simulink model "three_phase_topology"  (Simulink 8.5)
settings: Solver=ode45  StartTime=0.0  StopTime=10.0  MaxStep=0.0001  MinStep=0.00001  RelTol=1e-3
libraries: powerlib x37
settings Model: Creator=SELVA  LastModifiedBy=SELVA SAM  CovSFcnEnable=off
settings DataIOCC: SignalLoggingSaveFormat=Dataset
settings OptimizationCC: ExpressionDepthLimit=128
settings DebuggingCC: UnderspecifiedInitializationDetection=Simplified  MergeDetectMultiDrivingBlocksExec=error  SolverPrmCheckMsg=warning  FcnCallInpInsideContextMsg=EnableAllAsError  StateNameClashWarn=none
settings GRTTargetCC: CombineOutputUpdateFcns=on  GRTInterface=off
settings ConfigurationSet: Description=SimMechanics 2G

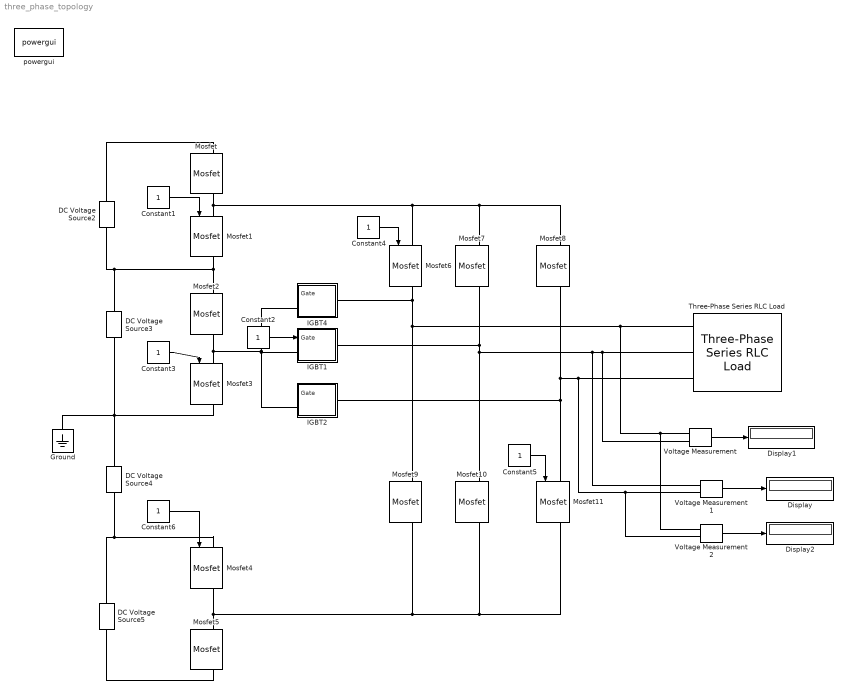
== system three_phase_topology ==
  Constant{1..6} (6 alike) : Constant
  DC Voltage Source{2..5} (4 alike) : powerlib/Electrical Sources/DC Voltage Source  Amplitude=600  Measurements=None
  Display : Display
  Display1 : Display
  Display2 : Display
  Ground : powerlib/Elements/Ground  LConnTagsString=a
  IGBT1 : Subsystem
  IGBT2 : Subsystem
  IGBT4 : Subsystem
  Mosfet{,1..11} (12 alike) : powerlib/Power Electronics/Mosfet  Ron=0.1  Lon=0  Rd=0.01  Vfd=0  IC=0  Rs=1e5  Cs=inf  Measurements=on
  Three-Phase Series RLC Load : powerlib/Elements/Three-Phase Series RLC Load  LConnTagsString=A|B|C  Configuration=Y (grounded)  NominalVoltage=400  NominalFrequency=50  ActivePower=1000  InductivePower=0  CapacitivePower=0  Measurements=None  LoadType=constant Z
  Voltage Measurement : powerlib/Measurements/Voltage Measurement  PhasorSimulation=off  OutputType=Complex  PSBequivalent=0
  Voltage Measurement1 : powerlib/Measurements/Voltage Measurement  PhasorSimulation=off  OutputType=Complex  PSBequivalent=0
  Voltage Measurement2 : powerlib/Measurements/Voltage Measurement  PhasorSimulation=off  OutputType=Complex  PSBequivalent=0
  powergui : powerlib/powergui  Priority=1  SimulationMode=Discrete  SolverType=Tustin/Backward Euler (TBE)  SampleTime=50e-6  frequency=60  SPID=off  DisableSnubberDevices=off  DisableRonSwitches=off  DisableVfSwitches=off  SwTol=0  DisplayEquations=off  Interpol=off  methode=off  Ts=100  frequencyindice=0  Pbase=100e6  ErrMax=1e-4  Iterations=50  UnitsV=kV  UnitsW=MW  FunctionMessages=off  echomessages=off  HookPort=off  EnableUseOfTLC=off  x0status=blocks  RestoreLinks=warning  ResistiveCurrentMeasurement=off  Frange=[0:2:500]  Ylog=off  Xlog=on  ShowGrid=off  save=off  variable=ZData  structure=0  ZoomFFT=off  StartTime=0.0  cycles=1  DisplayStyle=1  fundamental=60  FreqAxis=off  MaxFrequency=1000  frequencyindicesteady=1  RmsSteady=1  display=off
  wires:
  ? -> IGBT4/1(Gate)
  Constant2/1 -> IGBT1/1(Gate)
  ? -> IGBT2/1(Gate)
  Constant3/1 -> Mosfet3/1
  Constant4/1 -> Mosfet6/1
  Constant5/1 -> Mosfet11/1
  Constant1/1 -> Mosfet1/1
  Constant6/1 -> Mosfet4/1
  Voltage Measurement/1 -> Display1/1
  Voltage Measurement1/1 -> Display/1
  Voltage Measurement2/1 -> Display2/1
  connections:
  Mosfet3/LConn1 -- IGBT4/LConn1 -- IGBT2/LConn1 -- IGBT1/LConn1 -- Mosfet2/RConn1
  Mosfet2/LConn1 -- DC Voltage Source2/LConn1 -- DC Voltage Source3/RConn1 -- Mosfet1/RConn1
  DC Voltage Source2/RConn1 -- Mosfet/LConn1
  Ground/LConn1 -- DC Voltage Source4/RConn1 -- DC Voltage Source3/LConn1 -- Mosfet3/RConn1
  Mosfet4/LConn1 -- DC Voltage Source5/RConn1 -- DC Voltage Source4/LConn1
  Mosfet11/RConn1 -- Mosfet4/RConn1 -- Mosfet5/LConn1 -- Mosfet9/RConn1 -- Mosfet10/RConn1
  DC Voltage Source5/LConn1 -- Mosfet5/RConn1
  Mosfet11/LConn1 -- Voltage Measurement2/LConn2 -- Voltage Measurement1/LConn2 -- Three-Phase Series RLC Load/LConn3 -- Mosfet8/RConn1 -- IGBT2/RConn1
  Mosfet10/LConn1 -- Voltage Measurement1/LConn1 -- Voltage Measurement/LConn2 -- Three-Phase Series RLC Load/LConn2 -- Mosfet7/RConn1 -- IGBT1/RConn1
  Mosfet6/RConn1 -- Voltage Measurement2/LConn1 -- Voltage Measurement/LConn1 -- Three-Phase Series RLC Load/LConn1 -- Mosfet9/LConn1 -- IGBT4/RConn1
  Mosfet1/LConn1 -- Mosfet7/LConn1 -- Mosfet8/LConn1 -- Mosfet6/LConn1 -- Mosfet/RConn1

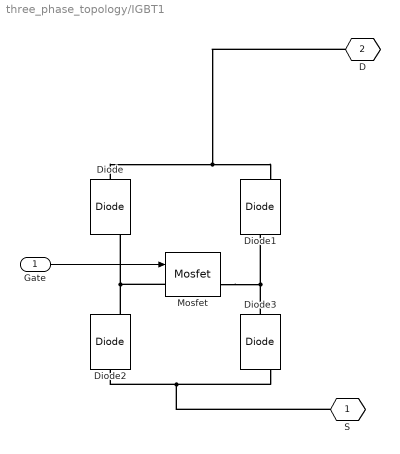
== system three_phase_topology/IGBT1 ==
  Gate : Inport
  Diode{,1..3} (4 alike) : powerlib/Power Electronics/Diode  Ron=0.001  Lon=0  Vf=0.8  IC=0  UseSnubber=off  Rs=500  Cs=250e-9  Measurements=on
  Mosfet : powerlib/Power Electronics/Mosfet  Ron=0.1  Lon=0  Rd=0.01  Vfd=0  IC=0  Rs=1e5  Cs=inf  Measurements=on
  S : PMIOPort  Port=1  Side=Left
  D : PMIOPort  Port=2  Side=Right
  wires:
  Gate/1 -> Mosfet/1
  connections:
  D/RConn1 -- Diode/LConn1 -- Diode1/RConn1
  S/RConn1 -- Diode3/RConn1 -- Diode2/LConn1
  Mosfet/RConn1 -- Diode3/LConn1 -- Diode1/LConn1
  Mosfet/LConn1 -- Diode2/RConn1 -- Diode/RConn1

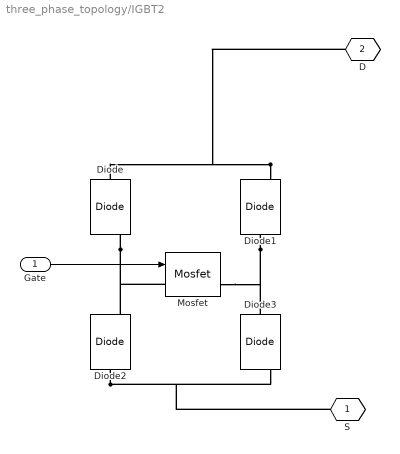
== system three_phase_topology/IGBT2 ==
  Gate : Inport
  Diode{,1..3} (4 alike) : powerlib/Power Electronics/Diode  Ron=0.001  Lon=0  Vf=0.8  IC=0  UseSnubber=off  Rs=500  Cs=250e-9  Measurements=on
  Mosfet : powerlib/Power Electronics/Mosfet  Ron=0.1  Lon=0  Rd=0.01  Vfd=0  IC=0  Rs=1e5  Cs=inf  Measurements=on
  S : PMIOPort  Port=1  Side=Left
  D : PMIOPort  Port=2  Side=Right
  wires:
  Gate/1 -> Mosfet/1
  connections:
  Diode/RConn1 -- Diode2/RConn1 -- Mosfet/LConn1
  Diode1/LConn1 -- Diode3/LConn1 -- Mosfet/RConn1
  Diode2/LConn1 -- Diode3/RConn1 -- S/RConn1
  Diode1/RConn1 -- Diode/LConn1 -- D/RConn1

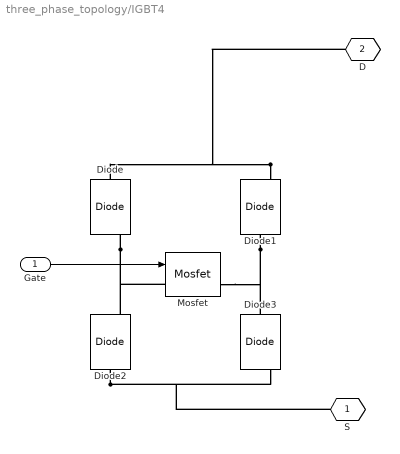
== system three_phase_topology/IGBT4 ==
  Gate : Inport
  Diode{,1..3} (4 alike) : powerlib/Power Electronics/Diode  Ron=0.001  Lon=0  Vf=0.8  IC=0  UseSnubber=off  Rs=500  Cs=250e-9  Measurements=on
  Mosfet : powerlib/Power Electronics/Mosfet  Ron=0.1  Lon=0  Rd=0.01  Vfd=0  IC=0  Rs=1e5  Cs=inf  Measurements=on
  S : PMIOPort  Port=1  Side=Left
  D : PMIOPort  Port=2  Side=Right
  wires:
  Gate/1 -> Mosfet/1
  connections:
  Diode/RConn1 -- Mosfet/LConn1 -- Diode2/RConn1
  Diode1/LConn1 -- Mosfet/RConn1 -- Diode3/LConn1
  Diode2/LConn1 -- Diode3/RConn1 -- S/RConn1
  Diode1/RConn1 -- Diode/LConn1 -- D/RConn1
